simulink model "Assignment2_2"  (R2020a)
settings: Solver=FixedStepAuto  StartTime=0.0  StopTime=10.0  FixedStep=1e-3  RelTol=1e-3  EnableMultiTasking=on
libraries: etargetslib x4, frdmk64flib x3
settings Model: ExtModeTrigDuration=5  Creator=iceca  LastModifiedBy=iceca
settings OptimizationCC: EnhancedBackFolding=on  PassReuseOutputArgsAs=Individual arguments  ZeroExternalMemoryAtStartup=off  ZeroInternalMemoryAtStartup=off  MaxStackSize=64  OptimizeBlockOrder=speed  DifferentSizesBufferReuse=on  OptimizationCustomize=off  EfficientTunableParamExpr=on
settings DebuggingCC: ParameterTunabilityLossMsg=error
settings HardwareCC: ProdBitPerPointer=32  ProdBitPerSizeT=32  ProdBitPerPtrDiffT=32  ProdLargestAtomicInteger=Long  ProdLargestAtomicFloat=Double  ProdWordSize=32  ProdHWDeviceType=ARM Compatible->ARM Cortex
settings SFSimCC: MATLABDynamicMemAlloc=off
settings RTWCC: SystemTargetFile=ert.tlc  HardwareBoard=NXP FRDM-K64F  TemplateMakefile=ert_default_tmf  Toolchain=GNU Tools for ARM Embedded Processors
settings CodeAppCC: ForceParamTrailComments=on  IgnoreCustomStorageClasses=off  OperatorAnnotations=on  SimulinkDataObjDesc=on  SFDataObjDesc=on  InsertBlockDesc=on

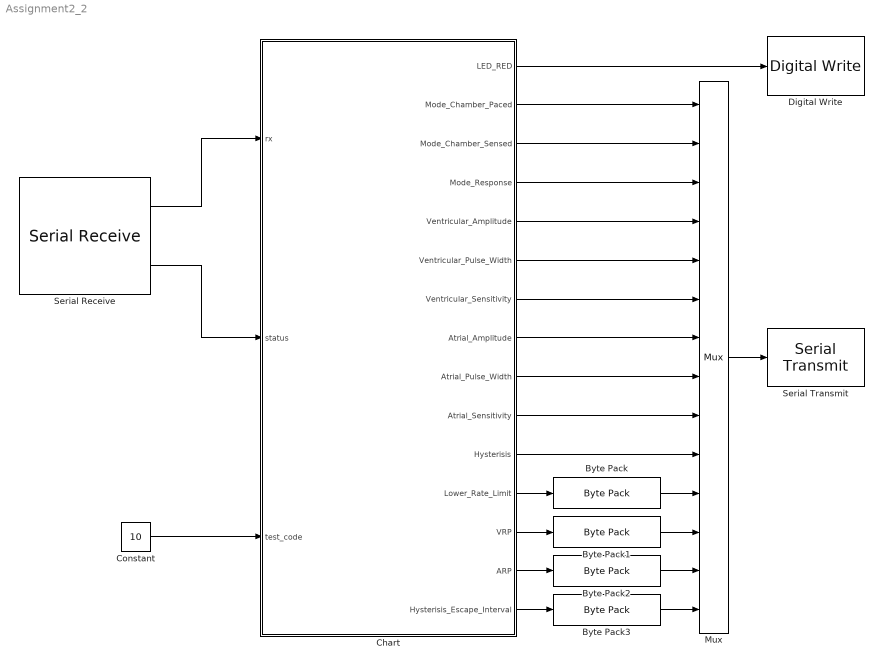
== system Assignment2_2 ==
  Byte Pack{,1..3} (4 alike) : etargetslib/Byte Pack  datatypes={'uint16'}  byteAlign=1
  Chart : Stateflow chart  TreatAsAtomicUnit=on
  Constant : Constant  Value=10
  Digital Write : frdmk64flib/Digital Write  Whichpin=RED_LED
  Mux : Mux  Inputs=14
  Serial Receive : frdmk64flib/Serial Receive  SCIModule=0  Baudrate=uint32(9600)  Parity=None  StopBits=1  HardwareFlowControl=None  ByteOrder=LittleEndian  DataType=uint8  DataLength=19  BlockingMode=off  OutputStatus=on  SampleTime=-1
  Serial Transmit : frdmk64flib/Serial Transmit  SCIModule=0  Baudrate=uint32(9600)  Parity=None  StopBits=1  HardwareFlowControl=None  ByteOrder=LittleEndian  BlockingMode=on  OutputStatus=off
  wires:
  Mux/1 -> Serial Transmit/1
  Serial Receive/1 -> Chart/1(rx)
  Serial Receive/2 -> Chart/2(status)
  Constant/1 -> Chart/3(test_code)
  Chart/1(LED_RED) -> Digital Write/1
  Chart/2(Mode_Chamber_Paced) -> Mux/1
  Chart/3(Mode_Chamber_Sensed) -> Mux/2
  Chart/4(Mode_Response) -> Mux/3
  Chart/5(Ventricular_Amplitude) -> Mux/4
  Chart/6(Ventricular_Pulse_Width) -> Mux/5
  Chart/7(Ventricular_Sensitivity) -> Mux/6
  Chart/8(Atrial_Amplitude) -> Mux/7
  Chart/9(Atrial_Pulse_Width) -> Mux/8
  Chart/10(Atrial_Sensitivity) -> Mux/9
  Chart/11(Hysterisis) -> Mux/10
  Chart/12(Lower_Rate_Limit) -> Byte Pack/1
  Byte Pack/1 -> Mux/11
  Byte Pack1/1 -> Mux/12
  Chart/13(VRP) -> Byte Pack1/1
  Byte Pack2/1 -> Mux/13
  Chart/14(ARP) -> Byte Pack2/1
  Chart/15(Hysterisis_Escape_Interval) -> Byte Pack3/1
  Byte Pack3/1 -> Mux/14

== stateflow chart Assignment2_2/Chart ==
  settings: executeAtInitialization=1
  state SET_UINT8
    entry:
    offset=2
    LED_RED =true;
    Mode_Chamber_Paced =  rx(offset);
    offset = offset + 1;
    Mode_Chamber_Sensed = rx(offset);
    offset = offset + 1;
    Mode_Response = rx(offset);
    offset = offset + 1;
    Ventricular_Amplitude = rx(offset);
    offset = offset + 1;
    Ventricular_Pulse_Width = rx(offset);
    offset = offset + 1;
    Ventricular_Sensitivity = rx(offset);
    offset = offset + 1;
    Atrial_Amplitude = rx(offset);
    offset = offset + 1;
    Atrial_Pulse_Width = rx(offset);
    offset = offset + 1;
    Atrial_Sensitivity = rx(offset);
    offset = offset + 1;
    Hysterisis =  rx(offset);
    offset = offset + 1;
    %a = typecast(rx(offset:offset+1),'uint16');
    %offset = offset+2;
    %b = rx(offset);
  state IDLE
    entry:
    LED_RED=false;
  state SET_UINT16
    entry:
    Lower_Rate_Limit = typecast(rx(offset:offset+1),'uint16');
    offset = offset+2;
    VRP = typecast(rx(offset:offset+1),'uint16');
    offset = offset+2;
    ARP = typecast(rx(offset:offset+1),'uint16');
    offset = offset+2;
    Hysterisis_Escape_Interval = typecast(rx(offset:offset+1),'uint16');
    offset = offset+2;
  (junction 11) -> SET_UINT8 [order 1] : [rx(1)==test_code]
  IDLE -> (junction 11) : [status==0]
  (junction 11) -> IDLE [order 2]
  (default) -> IDLE
  SET_UINT16 -> IDLE
  SET_UINT8 -> SET_UINT16
  data: rx input; status input; offset local; test_code input; LED_RED output; Mode_Chamber_Paced output; Mode_Chamber_Sensed output; Mode_Response output; Ventricular_Amplitude output; Ventricular_Pulse_Width output; Ventricular_Sensitivity output; Atrial_Amplitude output; Atrial_Pulse_Width output; Atrial_Sensitivity output; Hysterisis output; Lower_Rate_Limit output size=1; VRP output size=1; ARP output size=1; Hysterisis_Escape_Interval output size=1
